simulink model "curr_FF"  (R2013b)
settings: Solver=ode45  StartTime=0.0  StopTime=10.0  RelTol=1e-3
values from neighbouring files (symbols this model uses):
  pow = 1.88    [RunMotorSim.m]    (also in RunMotorSim_OpenLoop.m = 2)
settings Model: Creator=aberger  LastModifiedBy=aberger

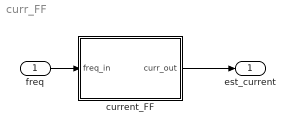
== system curr_FF ==
  freq : Inport
  current_FF : Subsystem
  est_current : Outport
  wires:
  freq/1 -> current_FF/1(freq_in)
  current_FF/1(curr_out) -> est_current/1

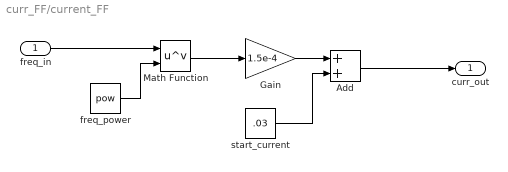
== system curr_FF/current_FF ==
  freq_in : Inport
  Add : Sum
  Gain : Gain  Gain=1.5e-4
  Math Function : Math  Operator=pow  SaturateOnIntegerOverflow=on
  freq_power : Constant  Value=pow
  start_current : Constant  Value=.03
  curr_out : Outport
  wires:
  Add/1 -> curr_out/1
  freq_power/1 -> Math Function/2
  Gain/1 -> Add/1
  start_current/1 -> Add/2
  freq_in/1 -> Math Function/1
  Math Function/1 -> Gain/1
